simulink model "lbdlp_simu"  (R2018a)
settings: Solver=FixedStepAuto  StartTime=0.0  StopTime=4  RelTol=1e-3
values from neighbouring files (symbols this model uses):
  A = eval(simplify(A))    [Bolita_2.m]    (also in Ej_parcial_2019.m = eval(A); les_boles_de_les_pibardes.m)
  B = eval(simplify(B))    [Bolita_2.m]    (also in Ej_parcial_2019.m = eval(B); les_boles_de_les_pibardes.m)
  C = [1, 0, 0]    [Bolita_2.m]    (also in Ej_parcial_2019.m = [1 0]; les_boles_de_les_pibardes.m)
  D = 0    [Bolita_2.m]    (also in Ej_parcial_2019.m; les_boles_de_les_pibardes.m)
  K = place(A, B, [-15 -3 -220])    [Bolita_2.m]    (also in les_boles_de_les_pibardes.m)
  Kic = Kai(4)    [Bolita_2.m]    (also in les_boles_de_les_pibardes.m)
  L = (acker(sysasd.A', sysasd.C', pDiscL))'    [Bolita_2.m]    (also in Ej_parcial_2019.m = place(Ad_obs',Cd_obs',[-10 -5]); les_boles_de_les_pibardes.m = (acker(A', C', [-160 -160 -160]))')
  Ts = 0.0001    [Bolita_2.m]    (also in Ej_parcial_2019.m = 0.1)
  x1 = double(x1_eq)    [Bolita_2.m]    (also in Ej_parcial_2019.m = 0; les_boles_de_les_pibardes.m)
  x2 = double(x2_eq)    [Bolita_2.m]    (also in Ej_parcial_2019.m = 0; les_boles_de_les_pibardes.m)
  x3 = double(x3_eq)    [Bolita_2.m]    (also in les_boles_de_les_pibardes.m)
undefined symbols (not defined in the file or in its folder): DiscIntNeverNeededParam
settings Model: Creator=Guido L  LastModifiedBy=Guido L

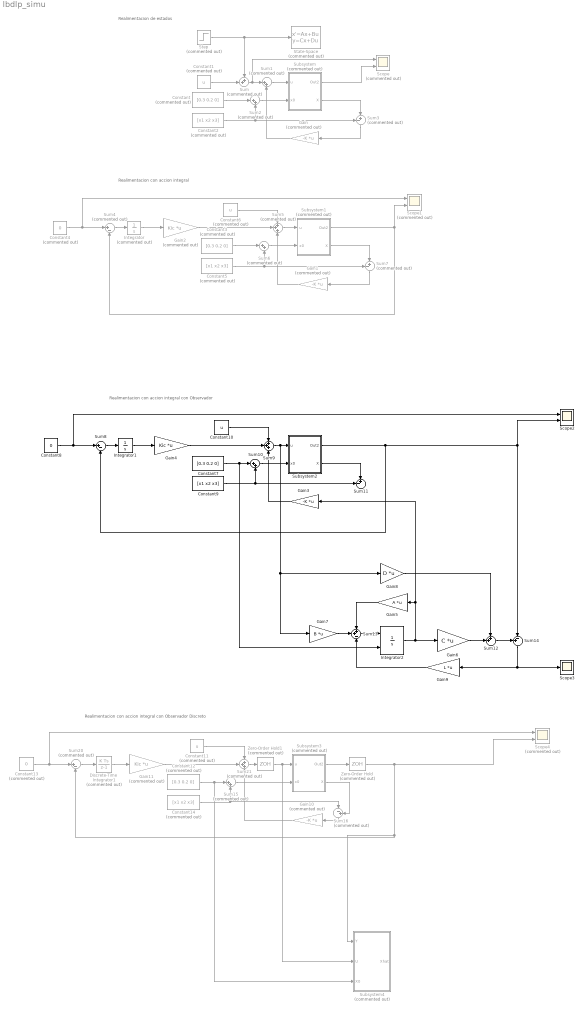
== system lbdlp_simu ==
  note: Realimentacion de estados
  note: Realimentacion con accion integral
  note: Realimentacion con accion integral con Observador
  note: Realimentacion con accion integral con Observador Discreto
  Constant : Constant  Commented=on  Value=[0.3 0.2 0]
  Constant1 : Constant  Commented=on  Value=u
  Constant10 : Constant  Value=u
  Constant11 : Constant  Commented=on  Value=u
  Constant12 : Constant  Commented=on  Value=[0.3 0.2 0]
  Constant13 : Constant  Commented=on  Value=0
  Constant14 : Constant  Commented=on  Value=[x1 x2 x3]
  Constant2 : Constant  Commented=on  Value=[x1 x2 x3]
  Constant3 : Constant  Commented=on  Value=[0.3 0.2 0]
  Constant4 : Constant  Commented=on  Value=0
  Constant5 : Constant  Commented=on  Value=[x1 x2 x3]
  Constant6 : Constant  Commented=on  Value=u
  Constant7 : Constant  Value=[0.3 0.2 0]
  Constant8 : Constant  Value=0
  Constant9 : Constant  Value=[x1 x2 x3]
  Discrete-Time Integrator1 : DiscreteIntegrator  Commented=on  SampleTime=Ts  ICPrevOutput=DiscIntNeverNeededParam  ICPrevScaledInput=DiscIntNeverNeededParam
  Gain : Gain  Commented=on  Gain=-K  Multiplication=Matrix(K*u) (u vector)
  Gain1 : Gain  Commented=on  Gain=-K  Multiplication=Matrix(K*u) (u vector)
  Gain10 : Gain  Commented=on  Gain=-K  Multiplication=Matrix(K*u) (u vector)
  Gain11 : Gain  Commented=on  Gain=Kic  Multiplication=Matrix(K*u) (u vector)
  Gain2 : Gain  Commented=on  Gain=Kic  Multiplication=Matrix(K*u) (u vector)
  Gain3 : Gain  Gain=-K  Multiplication=Matrix(K*u) (u vector)
  Gain4 : Gain  Gain=Kic  Multiplication=Matrix(K*u) (u vector)
  Gain5 : Gain  Gain=A  Multiplication=Matrix(K*u) (u vector)
  Gain6 : Gain  Gain=C  Multiplication=Matrix(K*u) (u vector)
  Gain7 : Gain  Gain=B  Multiplication=Matrix(K*u) (u vector)
  Gain8 : Gain  Gain=D  Multiplication=Matrix(K*u) (u vector)
  Gain9 : Gain  Gain=L  Multiplication=Matrix(K*u) (u vector)
  Integrator : Integrator  Commented=on
  Integrator1 : Integrator
  Integrator2 : Integrator  InitialConditionSource=external
  Scope : Scope  Commented=on  NumInputPorts=2
  Scope1 : Scope  Commented=on  NumInputPorts=2
  Scope2 : Scope  NumInputPorts=2
  Scope3 : Scope
  Scope4 : Scope  Commented=on  NumInputPorts=2
  State-Space : StateSpace  Commented=on  A=A  B=B  C=C  D=D  InitialCondition=0
  Step : Step  Commented=on  Time=0.1  After=0.08  SampleTime=0
  Subsystem : Subsystem  Commented=on
  Subsystem1 : Subsystem  Commented=on
  Subsystem2 : Subsystem
  Subsystem3 : Subsystem  Commented=on
  Subsystem4 : Subsystem  Commented=on
  Sum : Sum  Commented=on  Inputs=++|
  Sum{1..2,6,15} (4 alike) : Sum  Commented=on  Inputs=|++
  Sum10 : Sum  Inputs=|++
  Sum11 : Sum  Inputs=-+|
  Sum12 : Sum  Inputs=++|
  Sum13 : Sum  Inputs=++-
  Sum14 : Sum  Inputs=+-|
  Sum16 : Sum  Commented=on  Inputs=|-+
  Sum20 : Sum  Commented=on  Inputs=|+-
  Sum21 : Sum  Commented=on  Inputs=+++
  Sum3 : Sum  Commented=on  Inputs=-+|
  Sum4 : Sum  Commented=on  Inputs=|+-
  Sum5 : Sum  Commented=on  Inputs=+++
  Sum7 : Sum  Commented=on  Inputs=-+|
  Sum8 : Sum  Inputs=|+-
  Sum9 : Sum  Inputs=+++
  Zero-Order Hold : ZeroOrderHold  Commented=on  SampleTime=Ts
  Zero-Order Hold1 : ZeroOrderHold  Commented=on  SampleTime=Ts
  wires:
  Step/1 -> Sum/1, State-Space/1
  Subsystem/1(Out2) -> Scope/2
  Constant1/1 -> Sum/2
  Sum/1 -> Scope/1, Sum1/1
  Sum1/1 -> Subsystem/1(u)
  Gain/1 -> Sum1/2
  Subsystem/2(X) -> Sum3/2
  Sum3/1 -> Gain/1
  Constant2/1 -> Sum3/1, Sum2/2
  Constant/1 -> Sum2/1
  Sum2/1 -> Subsystem/2("x0 ")
  Subsystem1/1(Out2) -> Sum4/2, Scope1/2
  Constant5/1 -> Sum7/1, Sum6/2
  Sum6/1 -> Subsystem1/2("x0 ")
  Sum5/1 -> Subsystem1/1(u)
  Constant3/1 -> Sum6/1
  Sum7/1 -> Gain1/1
  Subsystem1/2(X) -> Sum7/2
  Constant4/1 -> Sum4/1, Scope1/1
  Integrator/1 -> Gain2/1
  Sum4/1 -> Integrator/1
  Gain2/1 -> Sum5/2
  Constant6/1 -> Sum5/1
  Gain1/1 -> Sum5/3
  Constant10/1 -> Sum9/1
  Gain4/1 -> Sum9/2
  Sum8/1 -> Integrator1/1
  Integrator1/1 -> Gain4/1
  Sum10/1 -> Subsystem2/2("x0 ")
  Constant7/1 -> Integrator2/2, Sum10/1
  Constant9/1 -> Sum11/1, Sum10/2
  Constant8/1 -> Sum8/1, Scope2/1
  Subsystem2/1(Out2) -> Scope2/2, Sum14/2, Sum8/2
  Gain3/1 -> Sum9/3
  Gain6/1 -> Sum12/2
  Gain8/1 -> Sum12/1
  Gain7/1 -> Sum13/2
  Gain5/1 -> Sum13/1
  Sum13/1 -> Integrator2/1
  Integrator2/1 -> Gain3/1, Gain5/1, Gain6/1
  Sum9/1 -> Gain7/1, Gain8/1, Subsystem2/1(u)
  Sum12/1 -> Sum14/1
  Gain9/1 -> Sum13/3
  Sum14/1 -> Scope3/1, Gain9/1
  Subsystem2/2(X) -> Sum11/2
  Constant13/1 -> Sum20/1, Scope4/1
  Constant14/1 -> Sum16/1, Sum15/2
  Sum15/1 -> Subsystem3/2("x0 ")
  Gain11/1 -> Sum21/2
  Discrete-Time Integrator1/1 -> Gain11/1
  Sum20/1 -> Discrete-Time Integrator1/1
  Constant11/1 -> Sum21/1
  Gain10/1 -> Sum21/3
  Subsystem3/1(Out2) -> Zero-Order Hold/1
  Zero-Order Hold/1 -> Scope4/2, Subsystem4/1(Y), Sum20/2
  Sum21/1 -> Zero-Order Hold1/1
  Subsystem3/2(X) -> Sum16/2
  Zero-Order Hold1/1 -> Subsystem4/2("U "), Subsystem3/1(u)
  Constant12/1 -> Subsystem4/3("X0 "), Sum15/1
  Sum16/1 -> Gain10/1

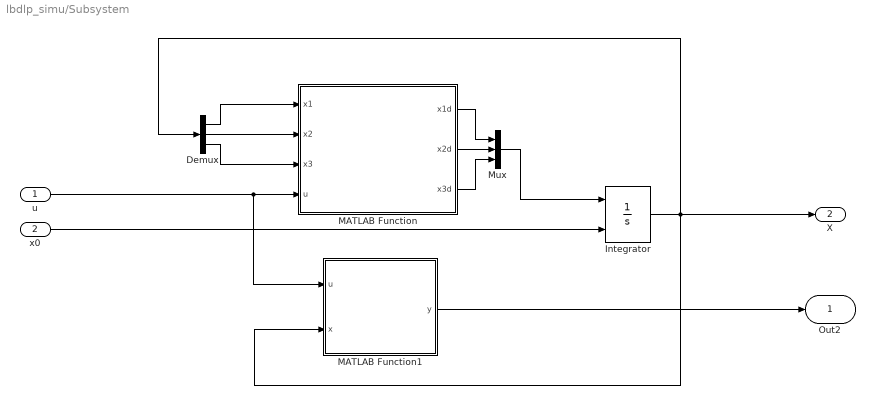
== system lbdlp_simu/Subsystem ==
  u : Inport
  "x0 " : Inport  Port=2
  Demux : Demux  Outputs=3
  Integrator : Integrator  InitialConditionSource=external
  MATLAB Function : MATLAB Function  TreatAsAtomicUnit=on
  MATLAB Function1 : MATLAB Function  TreatAsAtomicUnit=on
  Mux : Mux  Inputs=3
  Out2 : Outport
  X : Outport  Port=2
  wires:
  MATLAB Function/3(x3d) -> Mux/3
  Integrator/1 -> X/1, Demux/1, MATLAB Function1/2(x)
  MATLAB Function/1(x1d) -> Mux/1
  u/1 -> MATLAB Function1/1(u), MATLAB Function/4(u)
  Demux/1 -> MATLAB Function/1(x1)
  Demux/2 -> MATLAB Function/2(x2)
  MATLAB Function/2(x2d) -> Mux/2
  Mux/1 -> Integrator/1
  Demux/3 -> MATLAB Function/3(x3)
  MATLAB Function1/1(y) -> Out2/1
  "x0 "/1 -> Integrator/2

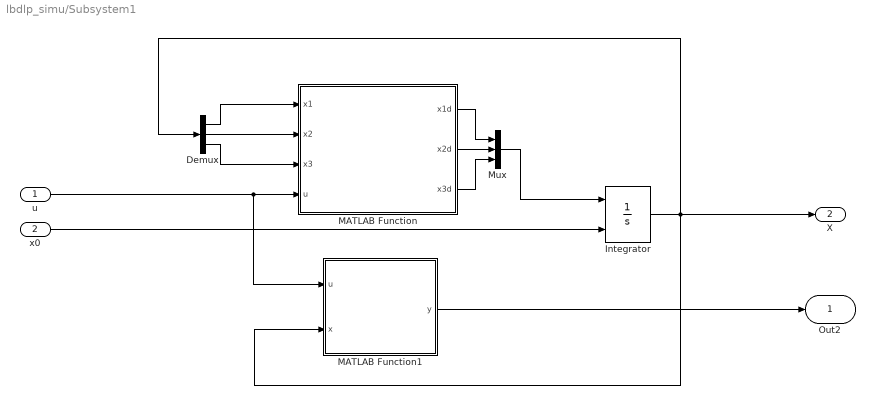
== system lbdlp_simu/Subsystem1 ==
  u : Inport
  "x0 " : Inport  Port=2
  Demux : Demux  Outputs=3
  Integrator : Integrator  InitialConditionSource=external
  MATLAB Function : MATLAB Function  TreatAsAtomicUnit=on
  MATLAB Function1 : MATLAB Function  TreatAsAtomicUnit=on
  Mux : Mux  Inputs=3
  Out2 : Outport
  X : Outport  Port=2
  wires:
  MATLAB Function/3(x3d) -> Mux/3
  Integrator/1 -> X/1, Demux/1, MATLAB Function1/2(x)
  MATLAB Function/1(x1d) -> Mux/1
  u/1 -> MATLAB Function1/1(u), MATLAB Function/4(u)
  Demux/1 -> MATLAB Function/1(x1)
  Demux/2 -> MATLAB Function/2(x2)
  MATLAB Function/2(x2d) -> Mux/2
  Mux/1 -> Integrator/1
  Demux/3 -> MATLAB Function/3(x3)
  MATLAB Function1/1(y) -> Out2/1
  "x0 "/1 -> Integrator/2

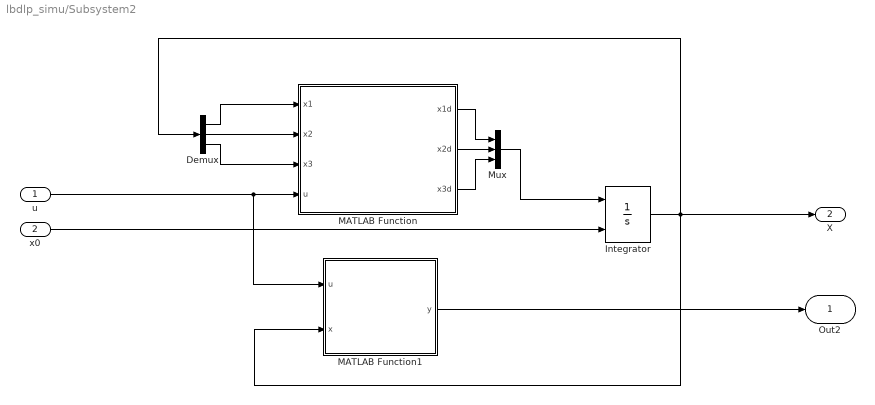
== system lbdlp_simu/Subsystem2 ==
  u : Inport
  "x0 " : Inport  Port=2
  Demux : Demux  Outputs=3
  Integrator : Integrator  InitialConditionSource=external
  MATLAB Function : MATLAB Function  TreatAsAtomicUnit=on
  MATLAB Function1 : MATLAB Function  TreatAsAtomicUnit=on
  Mux : Mux  Inputs=3
  Out2 : Outport
  X : Outport  Port=2
  wires:
  MATLAB Function/3(x3d) -> Mux/3
  Integrator/1 -> X/1, Demux/1, MATLAB Function1/2(x)
  MATLAB Function/1(x1d) -> Mux/1
  u/1 -> MATLAB Function1/1(u), MATLAB Function/4(u)
  Demux/1 -> MATLAB Function/1(x1)
  Demux/2 -> MATLAB Function/2(x2)
  MATLAB Function/2(x2d) -> Mux/2
  Mux/1 -> Integrator/1
  Demux/3 -> MATLAB Function/3(x3)
  MATLAB Function1/1(y) -> Out2/1
  "x0 "/1 -> Integrator/2

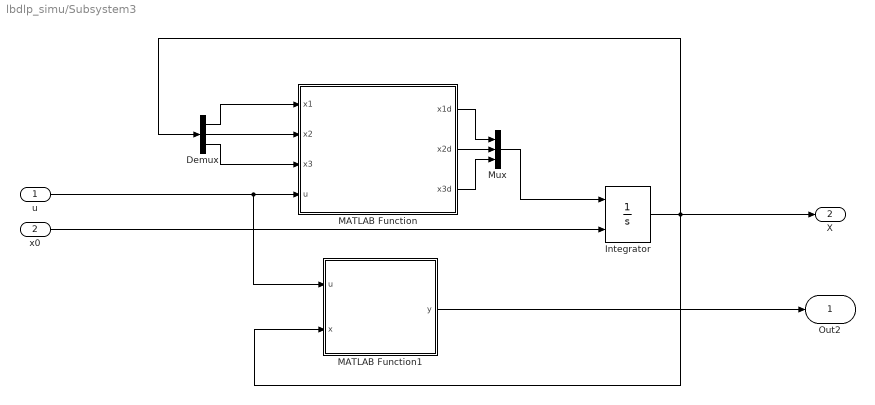
== system lbdlp_simu/Subsystem3 ==
  u : Inport
  "x0 " : Inport  Port=2
  Demux : Demux  Outputs=3
  Integrator : Integrator  InitialConditionSource=external
  MATLAB Function : MATLAB Function  TreatAsAtomicUnit=on
  MATLAB Function1 : MATLAB Function  TreatAsAtomicUnit=on
  Mux : Mux  Inputs=3
  Out2 : Outport
  X : Outport  Port=2
  wires:
  MATLAB Function/3(x3d) -> Mux/3
  Integrator/1 -> X/1, Demux/1, MATLAB Function1/2(x)
  MATLAB Function/1(x1d) -> Mux/1
  u/1 -> MATLAB Function1/1(u), MATLAB Function/4(u)
  Demux/1 -> MATLAB Function/1(x1)
  Demux/2 -> MATLAB Function/2(x2)
  MATLAB Function/2(x2d) -> Mux/2
  Mux/1 -> Integrator/1
  Demux/3 -> MATLAB Function/3(x3)
  MATLAB Function1/1(y) -> Out2/1
  "x0 "/1 -> Integrator/2

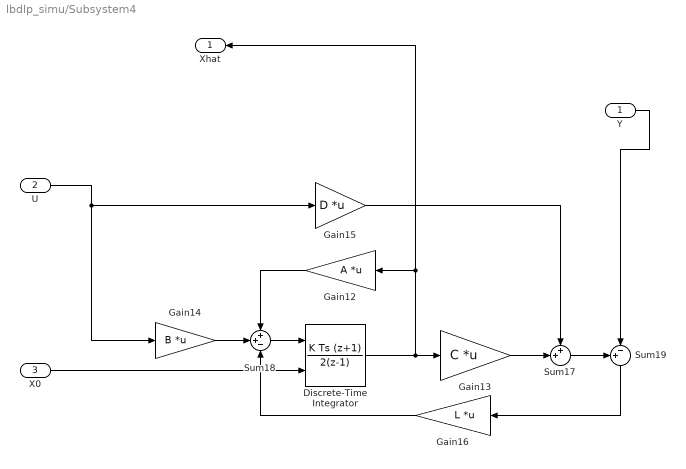
== system lbdlp_simu/Subsystem4 ==
  Y : Inport
  "U " : Inport  Port=2
  "X0 " : Inport  Port=3
  Discrete-Time Integrator : DiscreteIntegrator  IntegratorMethod=Integration: Trapezoidal  InitialConditionSource=external  SampleTime=Ts  ICPrevOutput=DiscIntNeverNeededParam  ICPrevScaledInput=DiscIntNeverNeededParam
  Gain12 : Gain  Gain=A  Multiplication=Matrix(K*u) (u vector)
  Gain13 : Gain  Gain=C  Multiplication=Matrix(K*u) (u vector)
  Gain14 : Gain  Gain=B  Multiplication=Matrix(K*u) (u vector)
  Gain15 : Gain  Gain=D  Multiplication=Matrix(K*u) (u vector)
  Gain16 : Gain  Gain=L  Multiplication=Matrix(K*u) (u vector)
  Sum17 : Sum  Inputs=++|
  Sum18 : Sum  Inputs=++-
  Sum19 : Sum  Inputs=+-|
  "Xhat " : Outport
  wires:
  Discrete-Time Integrator/1 -> "Xhat "/1, Gain12/1, Gain13/1
  Sum17/1 -> Sum19/1
  Gain13/1 -> Sum17/2
  Gain16/1 -> Sum18/3
  Sum19/1 -> Gain16/1
  Sum18/1 -> Discrete-Time Integrator/1
  "U "/1 -> Gain15/1, Gain14/1
  Gain15/1 -> Sum17/1
  Gain14/1 -> Sum18/2
  Gain12/1 -> Sum18/1
  "X0 "/1 -> Discrete-Time Integrator/2
  Y/1 -> Sum19/2

== matlab function lbdlp_simu/Subsystem/MATLAB Function1 ==
  data: u input; x input; y output
function y = fcn(u, x)
y = x(1);

== matlab function lbdlp_simu/Subsystem/MATLAB Function ==
  data: x1 input; x2 input; x3 input; u input; x1d output; x2d output; x3d output
function [x1d, x2d, x3d] = fcn(x1, x2, x3, u)

    g=10;
    m=0.2;
    L=1;
    R=4;
    
    f1 = 0.5*(2+x3)^2/(1-x1)^2;
    f2 = 0.5*(2-x3)^2/(1+x1)^2;
        
    x1d = x2;
    x2d = -g + f1/m - f2/m;
    x3d = -abs(x3)*x3*R/L+u/L;

== matlab function lbdlp_simu/Subsystem1/MATLAB Function ==
  data: x1 input; x2 input; x3 input; u input; x1d output; x2d output; x3d output
function [x1d, x2d, x3d] = fcn(x1, x2, x3, u)

    g=10;
    m=0.2;
    L=1;
    R=4;
    
    f1 = 0.5*(2+x3)^2/(1-x1)^2;
    f2 = 0.5*(2-x3)^2/(1+x1)^2;
        
    x1d = x2;
    x2d = -g + f1/m - f2/m;
    x3d = -abs(x3)*x3*R/L+u/L;

== matlab function lbdlp_simu/Subsystem1/MATLAB Function1 ==
  data: u input; x input; y output
function y = fcn(u, x)
y = x(1);

== matlab function lbdlp_simu/Subsystem2/MATLAB Function ==
  data: x1 input; x2 input; x3 input; u input; x1d output; x2d output; x3d output
function [x1d, x2d, x3d] = fcn(x1, x2, x3, u)

    g=10;
    m=0.2;
    L=1;
    R=4;
    
    f1 = 0.5*(2+x3)^2/(1-x1)^2;
    f2 = 0.5*(2-x3)^2/(1+x1)^2;
        
    x1d = x2;
    x2d = -g + f1/m - f2/m;
    x3d = -abs(x3)*x3*R/L+u/L;

== matlab function lbdlp_simu/Subsystem2/MATLAB Function1 ==
  data: u input; x input; y output
function y = fcn(u, x)
y = x(1);

== matlab function lbdlp_simu/Subsystem3/MATLAB Function ==
  data: x1 input; x2 input; x3 input; u input; x1d output; x2d output; x3d output
function [x1d, x2d, x3d] = fcn(x1, x2, x3, u)

    g=10;
    m=0.2;
    L=1;
    R=4;
    
    f1 = 0.5*(2+x3)^2/(1-x1)^2;
    f2 = 0.5*(2-x3)^2/(1+x1)^2;
        
    x1d = x2;
    x2d = -g + f1/m - f2/m;
    x3d = -abs(x3)*x3*R/L+u/L;

== matlab function lbdlp_simu/Subsystem3/MATLAB Function1 ==
  data: u input; x input; y output
function y = fcn(u, x)
y = x(1);
